simulink model "AEBTestBench"  (R2022b)
settings: Solver=ode45  StartTime=0.0  StopTime=inf  FixedStep=0.05  RelTol=1e-3
PostLoadFcn:
  | helperSLAEBSetup()
model workspace (MAT data in the model file):
  scenario : drivingScenario (value not decoded)
values from neighbouring files (symbols this model uses):
  actorsProfiles = rmfield(actorsProfiles,'MeshFaces')    [helperSLAEBSetup.m]
  egoActorID = egoVehicle.ActorID    [helperSLAEBSetup.m]
  egoRefPath = helperEgoRefPathCreator(scenario, egoActorID)    [helperSLAEBSetup.m]
  Ts = 0.05    [helperSLAEBSetup.m]
  v_set = norm(egoVehicle.Velocity)    [helperSLAEBSetup.m]
undefined symbols (not defined in the file or in its folder): cameraParams, driving, matlabshared, radarParams
libraries: drivingscenarioandsensors x3, simulink x2
CloseFcn:
  | helperSLAEBCleanup
settings Model: SILPILSystemUnderTest=refmodels  SnapshotInterval=5  PacingRate=0.220000  Creator=The MathWorks, Inc.  LastModifiedBy=yunuo
settings SolverCC: AlgebraicLoopSolver=TrustRegion  MinimalZcImpactIntegration=on  MaxZcPerStep=1
settings DataIOCC: SaveTime=off  ReturnWorkspaceOutputs=off
settings OptimizationCC: DefaultParameterBehavior=Inlined  InlineInvariantSignals=on  PassReuseOutputArgsAs=Individual arguments  ZeroExternalMemoryAtStartup=off  OptimizeBlockOrder=speed  EfficientTunableParamExpr=on
settings DebuggingCC: ParameterTunabilityLossMsg=error  UnconnectedInputMsg=warning  UnconnectedOutputMsg=warning  UnconnectedLineMsg=warning  PregeneratedLibrarySubsystemCodeDiagnostic=none  SFMachineParentedDataDiag=warning  ArithmeticOperatorsInVariantConditions=warning
settings HardwareCC: ProdLongLongMode=on
settings ModelReferenceCC: EnableRefExpFcnMdlSchedulingChecks=on  ModelReferenceNumInstancesAllowed=Single  PropagateVarSize=Only when enabling
settings SFSimCC: SimUseLocalCustomCode=off  CustomCodeUndefinedFunction=UseInterfaceOnly
settings RTWCC: Description=Embedded Coder  SystemTargetFile=ert.tlc  TemplateMakefile=ert_default_tmf  GenerateReport=on  RTWUseLocalCustomCode=off  BuildConfiguration=Faster Runs  IncludeHyperlinkInReport=on  LaunchReport=on  GenerateTraceInfo=on  GenerateTraceReport=on  GenerateTraceReportSl=on  GenerateTraceReportSf=on  GenerateTraceReportEml=on  GenerateCodeMetricsReport=on  DLArmComputeVersion=19.05
settings CodeAppCC: ForceParamTrailComments=on  IgnoreCustomStorageClasses=off  OperatorAnnotations=on  SimulinkDataObjDesc=on  SFDataObjDesc=on  CustomSymbolStrFcn=$N$M$F  InsertBlockDesc=on
settings ERTTargetCC: TargetLangStandard=C99 (ISO)  GenerateSampleERTMain=on  CombineSignalStateStructs=on  SuppressErrorStatus=on  InlinedParameterPlacement=NonHierarchical  RootIOFormat=Structure reference  RTWCAPISignals=on  ERTCustomFileTemplate=example_file_process.tlc

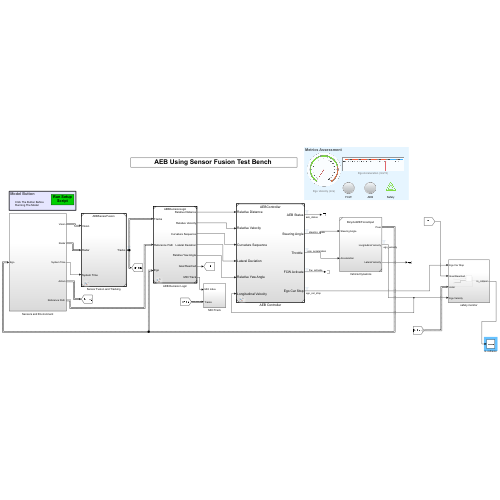
[thumbnail: Simulink's stored preview of the top-level diagram]
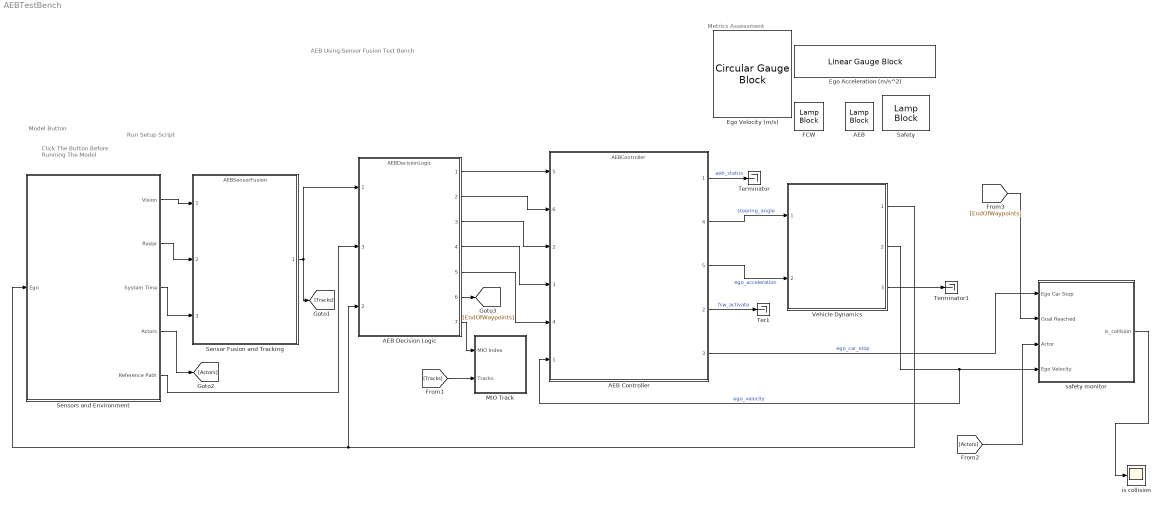
== system AEBTestBench ==
  note: Click The Button Before Running The Model
  note: Model Button
  note: AEB Using Sensor Fusion Test Bench
  note: Run Setup Script
  note: Metrics Assessment
  AEB : LampBlock  LabelPosition=Hide
  AEB Controller : ModelReference  ModelNameDialog=AEBController.slx  SimulationMode=Normal  CodeInterface=Top model  ModelReferenceVersion=5.0
      settings: PortSchema="{\"entries\":[{\"content\":{\"sides\":[{\"content\":{\"connectorIds\":[\"In5\",\"In6\",\"In2\",\"In3\",\"In4\",\"In1\"]},\"type\":\"ConnectorPlacement.EquallySpacedRectSide\",\"uuid\":\"48eb62e1-c687-4ccc-af1d-5db323c86b02\"},{\"content\":{\"connectorIds\":[\"Out1\",\"Out4\",\"Out5\",\"Out2\",\"Out3\"],\"side\":\"RIGHT\"},\"type\":\"ConnectorPlacement.EquallySpacedRectSide\",\"uuid\":\"cf0b79c1-cc3c-4144-ab0a-ade48c99ebae\"},{\"content\":{\"connectorIds\":[],\"side\":\"TOP\"},\"type\":\"ConnectorPlacement.EquallySpacedRectSide\",\"uuid\":\"b5029296-17a7-4a3b-9030-50c7482e3f67\"}]},\"type\":\"ConnectorPlacement.EquallySpacedConnector\",\"uuid\":\"17fe6146-247b-40c2-bc98-b1cbe9fc8f16\"}],\"packageUris\":[\"http://schema.mathworks.com/mf0/Connector/R2020b\"],\"version\":\"1.0\"}"
  AEB Decision Logic : ModelReference  ModelNameDialog=AEBDecisionLogic.slx  SimulationMode=Normal  CodeInterface=Top model  ModelReferenceVersion=5.1
      settings: PortSchema="{\"entries\":[{\"content\":{\"sides\":[{\"content\":{\"connectorIds\":[\"In1\",\"In3\",\"In2\"]},\"type\":\"ConnectorPlacement.EquallySpacedRectSide\",\"uuid\":\"e56e8f8b-a309-4236-958d-7c071b30483d\"},{\"content\":{\"connectorIds\":[\"Out1\",\"Out2\",\"Out3\",\"Out4\",\"Out5\",\"Out6\",\"Out7\"],\"side\":\"RIGHT\"},\"type\":\"ConnectorPlacement.EquallySpacedRectSide\",\"uuid\":\"786f45c2-22a8-47c8-9611-adc89b05d8ab\"},{\"content\":{\"connectorIds\":[],\"side\":\"TOP\"},\"type\":\"ConnectorPlacement.EquallySpacedRectSide\",\"uuid\":\"5bf649b4-ba14-4001-82ca-fb4560d0e6eb\"}]},\"type\":\"ConnectorPlacement.EquallySpacedConnector\",\"uuid\":\"abe3d890-2016-4578-afe8-a79cce07cd81\"}],\"packageUris\":[\"http://schema.mathworks.com/mf0/Connector/R2020b\"],\"version\":\"1.0\"}"
  Ego Acceleration (m/s^2) : LinearGaugeBlock  LabelPosition=Hide  ScaleMin=-9.8  ScaleMax=3  TickInterval=1
  Ego Velocity (m/s) : CircularGaugeBlock  LabelPosition=Hide  ScaleMax=20
  FCW : LampBlock  LabelPosition=Hide
  MIO Track : Subsystem
  Safety : LampBlock  LabelPosition=Hide  Icon=Hazards
  Sensor Fusion and Tracking : ModelReference  ModelNameDialog=AEBSensorFusion.slx  SimulationMode=Normal  CodeInterface=Top model  ModelReferenceVersion=5.2
  Sensors and Environment : Subsystem
  Ter1 : Terminator
  Terminator : Terminator
  Terminator1 : Terminator
  Vehicle Dynamics : Subsystem  ReferencedSubsystem=BicycleWithForceInput
  is collision : Scope
  safety monitor : Subsystem
  wires:
  AEB Controller/1 -> Terminator/1  "aeb_status"
  AEB Controller/2 -> Ter1/1  "fcw_activate"
  Vehicle Dynamics/1 -> Sensors and Environment/1(Ego), AEB Decision Logic/2
  Sensors and Environment/2(Radar) -> Sensor Fusion and Tracking/2
  Sensor Fusion and Tracking/1 -> AEB Decision Logic/1, [Tracks]
  Sensors and Environment/3(System Time) -> Sensor Fusion and Tracking/3
  Sensors and Environment/1(Vision) -> Sensor Fusion and Tracking/1
  AEB Decision Logic/5 -> AEB Controller/4
  AEB Decision Logic/4 -> AEB Controller/3
  AEB Decision Logic/3 -> AEB Controller/2
  AEB Decision Logic/1 -> AEB Controller/5
  AEB Decision Logic/2 -> AEB Controller/6
  AEB Decision Logic/6 -> [EndOfWaypoints]
  Sensors and Environment/4(Actors) -> [Actors]
  [Tracks] -> MIO Track/2(Tracks)
  AEB Decision Logic/7 -> MIO Track/1(MIO Index)
  Vehicle Dynamics/3 -> Terminator1/1
  AEB Controller/5 -> Vehicle Dynamics/2  "ego_acceleration"
  AEB Controller/4 -> Vehicle Dynamics/1  "steering_angle"
  Sensors and Environment/5("Reference Path ") -> AEB Decision Logic/3
  [Actors] -> safety monitor/3(Actor)
  [EndOfWaypoints] -> safety monitor/2(Goal Reached)
  AEB Controller/3 -> safety monitor/1(Ego Car Stop)  "ego_car_stop"
  Vehicle Dynamics/2 -> AEB Controller/1, safety monitor/4(Ego Velocity)  "ego_velocity"
  safety monitor/1(is_collision) -> is collision/1

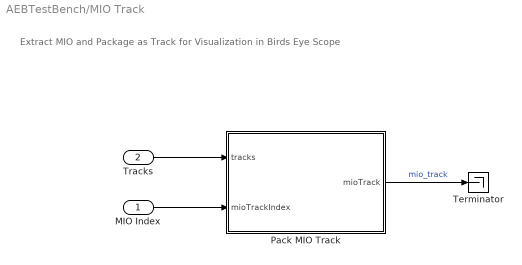
== system AEBTestBench/MIO Track ==
  note: Extract MIO and Package as Track for Visualization in Birds Eye Scope
  MIO Index : Inport
  Tracks : Inport  Port=2
  Pack MIO Track : MATLAB Function  TreatAsAtomicUnit=on
  Terminator : Terminator
  wires:
  Pack MIO Track/1(mioTrack) -> Terminator/1  "mio_track"
  Tracks/1 -> Pack MIO Track/1(tracks)
  MIO Index/1 -> Pack MIO Track/2(mioTrackIndex)

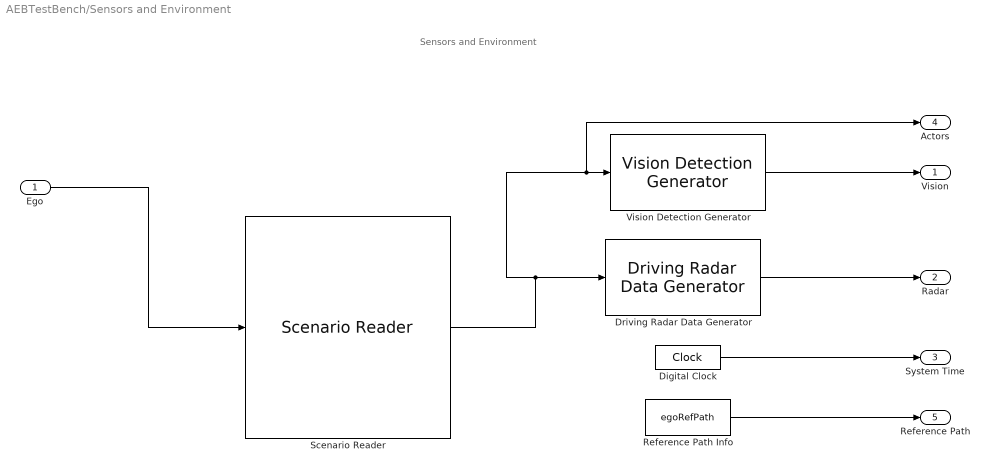
== system AEBTestBench/Sensors and Environment ==
  note: Sensors and Environment
  Ego : Inport
  Digital Clock : DigitalClock  SampleTime=Ts
  Driving Radar Data Generator : drivingscenarioandsensors/Driving Radar Data Generator  SensorIndex=2  UpdateRate=1/Ts  MountingLocation=[ 3.7, 0, 0.2 ]  MountingAngles=[0 0 0]  HasElevation=off  HasRangeRate=on  HasNoise=on  HasFalseAlarms=on  HasOcclusion=on  MaxNumReportsSource=Property  MaxNumReports=50  TargetReportFormat=Clustered detections  DetectionCoordinates=Body  TrackCoordinates=Body  BusNameSource=Property  BusName=BusRadar  AzimuthResolution=radarParams.azRes  ElevationResolution=5  RangeResolution=radarParams.rangeRes  RangeRateResolution=radarParams.rangeRateRes  AzimuthBiasFraction=0.1  ElevationBiasFraction=0.1  RangeBiasFraction=0.05  RangeRateBiasFraction=0.05  FieldOfView=[ radarParams.azFov, 5 ]  RangeLimits=[ 0, radarParams.radarRange ]  RangeRateLimits=[ -100, 100 ]  DetectionProbability=0.9  FalseAlarmRate=1e-06  ReferenceRange=100  ReferenceRCS=0  CenterFrequency=77e9  FilterInitializationFcn=initcvekf  ConfirmationThreshold=[2 3]  DeletionThreshold=[5 5]  InitialSeedSource=Repeatable  InitialSeed=0  UsedSeed=matlabshared.tracking.internal.SimulinkUtilities.seedManager(gcb)  ProfilesSource=From Scenario Reader block  ProfilesParameters=driving.internal.ActorProfilesRadarParameters  ProfilesExpression=struct('ClassID',0,'Length',4.7,'Width',1.8,'Height',1.4,'OriginOffset',[-1.35 0 0],'RCSPattern',[10 10;10 10],'RCSAzimuthAngles',[-180 180],'RCSElevationAngles',[-90 90])
  Reference Path Info : Constant  Value=egoRefPath  OutDataTypeStr=Bus: BusEgoRefPath  SampleTime=Ts
  Scenario Reader : drivingscenarioandsensors/Scenario Reader  ScenarioSource=From workspace  ScenarioFileName=AEB_CCRs_100overlap.mat  ScenarioVariableName=scenario  OutputCoordinateSystem=Vehicle coordinates  EgoVehicleSource=Input port  EgoVehicleActorID=egoActorID  OrientVehiclesOnRoad=on  OutputEgoVehiclePose=off  OutputEgoVehicleState=off  SampleTime=Ts  LaneBoundaryOutput=None  LaneBoundaryDistance=0:0.5:9.5  LaneBoundaryLocation=Center of lane markings  BusNameSource=Auto  BusName=BusActors  BusNumActorsSource=Scenario  BusNumActors=100  BusName2Source=Auto  BusName2=BusLaneBoundaries  BusNumLaneBoundariesSource=Scenario  BusNumLaneBoundaries=10  BusName3Source=Auto  BusName3=BusEgoActor  BusName4Source=Auto  BusName4=BusEgoState  ShowCoordinateLabels=on  SimulateUsing=Interpreted execution
  Vision Detection Generator : drivingscenarioandsensors/Vision Detection Generator  SensorIndex=1  DetectorOutput=Objects only  UpdateInterval=Ts  LaneUpdateInterval=Ts  SensorLocation=[ 2.1, 0 ]  Height=1.1  Yaw=0  Pitch=cameraParams.pitchAngle  Roll=0  BusNameSource=Property  BusName=BusVision  BusName2Source=Auto  BusName2=BusLaneDetections  MaxNumDetectionsSource=Property  MaxNumDetections=20  MaxNumLanesSource=Property  MaxNumLanes=30  DetectionCoordinates=Ego Cartesian  SimulateUsing=Interpreted execution  MaxRange=cameraParams.cameraRange  BoundingBoxAccuracy=5  ProcessNoiseIntensity=5  MaxSpeed=50  MaxAllowedOcclusion=0.5  MinObjectImageSize=[ 15, 15 ]  DetectionProbability=0.9  FalsePositivesPerImage=0.1  MinLaneImageSize=[ 20, 5 ]  LaneBoundaryAccuracy=3  HasNoise=on  InitialSeedSource=Repeatable  InitialSeed=0  UsedSeed=driving.internal.SimulinkUtilities.seedManager(gcb)  ActorProfilesSource=From Scenario Reader block  ActorProfilesParameters=driving.internal.ActorProfilesParameters  ActorProfilesExpression=struct( 'ClassID', 0, 'Length', 4.7, 'Width', 1.8, 'Height', 1.4, 'OriginOffset', [ -1.35, 0, 0 ] )  Intrinsics=driving.internal.cameraIntrinsics('FocalLength',cameraParams.focalLength,'PrincipalPoint',cameraParams.principalPoint,'ImageSize',cameraParams.imageSize)
  Vision : Outport  VectorParamsAs1DForOutWhenUnconnected=off
  Radar : Outport  Port=2  OutDataTypeStr=Bus: BusRadar  VectorParamsAs1DForOutWhenUnconnected=off
  System Time : Outport  Port=3  VectorParamsAs1DForOutWhenUnconnected=off
  Actors : Outport  Port=4
  "Reference Path " : Outport  Port=5
  wires:
  Vision Detection Generator/1 -> Vision/1
  Ego/1 -> Scenario Reader/1
  Digital Clock/1 -> System Time/1
  Driving Radar Data Generator/1 -> Radar/1
  Scenario Reader/1 -> Actors/1, Vision Detection Generator/1, Driving Radar Data Generator/1
  Reference Path Info/1 -> "Reference Path "/1

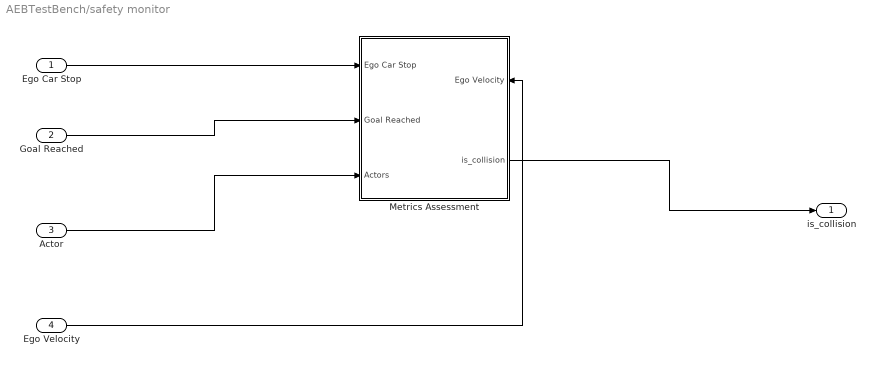
== system AEBTestBench/safety monitor ==
  Ego Car Stop : Inport
  Goal Reached : Inport  Port=2
  Actor : Inport  Port=3
  Ego Velocity : Inport  Port=4
  Metrics Assessment : Subsystem
      settings: PortSchema="{\"entries\":[{\"content\":{\"sides\":[{\"content\":{\"connectorIds\":[\"In1\",\"In2\",\"In3\"]},\"type\":\"ConnectorPlacement.EquallySpacedRectSide\",\"uuid\":\"d600d027-9714-4589-bd74-ff85c373770c\"},{\"content\":{\"connectorIds\":[\"In4\",\"Out1\"],\"side\":\"RIGHT\"},\"type\":\"ConnectorPlacement.EquallySpacedRectSide\",\"uuid\":\"c68a0d3a-3a81-49cd-ba70-f2de3f1a882f\"},{\"content\":{\"connectorIds\":[],\"side\":\"TOP\"},\"type\":\"ConnectorPlacement.EquallySpacedRectSide\",\"uuid\":\"d9b15fac-7ed3-4474-96f3-d7b693286234\"},{\"content\":{\"connectorIds\":[],\"side\":\"BOTTOM\"},\"type\":\"ConnectorPlacement.EquallySpacedRectSide\",\"uuid\":\"00c5a332-b546-4dc5-aa31-259f1868ab67\"}]},\"type\":\"ConnectorPlacement.EquallySpacedConnector\",\"uuid\":\"e6d068d7-d2df-4de9-99aa-2a189a2c2730\"}],\"packageUris\":[\"http://schema.mathworks.com/mf0/Connector/R2020b\"],\"version\":\"1.0\"}"
  is_collision : Outport
  wires:
  Ego Car Stop/1 -> Metrics Assessment/1(Ego Car Stop)
  Goal Reached/1 -> Metrics Assessment/2(Goal Reached)
  Actor/1 -> Metrics Assessment/3(Actors)
  Ego Velocity/1 -> Metrics Assessment/4(Ego Velocity)
  Metrics Assessment/1(is_collision) -> is_collision/1

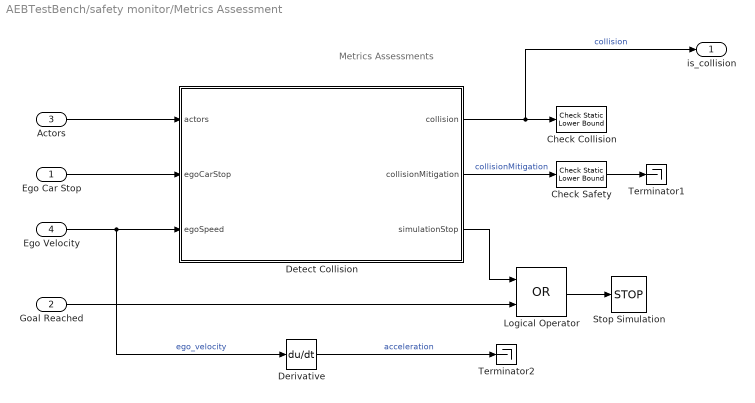
== system AEBTestBench/safety monitor/Metrics Assessment ==
  note: Metrics Assessments
  Ego Car Stop : Inport
  Goal Reached : Inport  Port=2
  Actors : Inport  Port=3
  Ego Velocity : Inport  Port=4
  Check Collision : simulink/Model Verification/Check Static  Lower Bound  Description=0 <= u  min=0  min_included=on  enabled=on  stopWhenAssertionFail=off  export=off  icon=graphic
  Check Safety : simulink/Model Verification/Check Static  Lower Bound  Description=safetyGoal <= u  min=safetyGoal  min_included=on  enabled=on  stopWhenAssertionFail=off  export=on  icon=graphic
  Derivative : Derivative
  Detect Collision : MATLAB Function  TreatAsAtomicUnit=on  mask(Detect Collision){vehicleProfiles=actorsProfiles, setSpeed=v_set, egoActorID=egoActorID}
      mask prompts: vehicleProfiles "Vehicle profiles"; setSpeed "Set Speed"; egoActorID "Ego Actor ID"
      mask help:
      | Detect collision between ego and target vehicles.
      | Vehicle profiles is expected to be the struture returned by the actorProfiles method of a drivingScenerio object.
      settings: AttributesFormatString=|
      | ------------------------------------------
      | vehicleProfiles = %<vehicleProfiles>
  Logical Operator : Logic  Operator=OR  AllPortsSameDT=off  OutDataTypeStr=boolean
  Stop Simulation : Stop
  Terminator1 : Terminator
  Terminator2 : Terminator
  is_collision : Outport
  wires:
  Ego Car Stop/1 -> Detect Collision/2(egoCarStop)
  Derivative/1 -> Terminator2/1  "acceleration"
  Ego Velocity/1 -> Derivative/1, Detect Collision/3(egoSpeed)  "ego_velocity"
  Actors/1 -> Detect Collision/1(actors)
  Detect Collision/1(collision) -> is_collision/1, Check Collision/1  "collision"
  Detect Collision/2(collisionMitigation) -> Check Safety/1  "collisionMitigation"
  Goal Reached/1 -> Logical Operator/2
  Logical Operator/1 -> Stop Simulation/1
  Detect Collision/3(simulationStop) -> Logical Operator/1
  Check Safety/1 -> Terminator1/1

== matlab function AEBTestBench/safety monitor/Metrics Assessment/Detect Collision ==
  data: actors input; collision output; vehicleProfiles parameter; egoCarStop input; collisionMitigation output; simulationStop output; setSpeed parameter; egoSpeed input double; egoActorID parameter
function [collision, collisionMitigation, simulationStop] = detectCollision(actors, vehicleProfiles, egoCarStop, setSpeed, egoSpeed, egoActorID)

% Associate on-path MATLAB function
coder.extrinsic('helperSLDetectVehicleCollision', 'warning');

% Assign default value to define output data type
collision = false;

% Call on-path MATLAB function
collision = helperSLDetectVehicleCollision(actors.Actors, vehicleProfiles, egoActorID = egoActorID);

if egoCarStop==true && collision==false
    collisionMitigation = 100.0; % Full collision avoidance = 100% collision migitation
elseif collision==true % collision detection
    collisionMitigation  = 100*(setSpeed-egoSpeed)/setSpeed; % calculate collision migitation
else
    collisionMitigation = 100.0; % neither collision nor ego car stop
end 

% if collision==true
%    error('Simulation stopped because of collision');
% end

if egoCarStop==true || collision==true
    simulationStop = true;
else
    simulationStop = false;
end

== matlab function AEBTestBench/MIO Track/Pack MIO Track ==
  data: tracks input; mioTrack output Bus: BusMultiObjectTracker1; mioTrackIndex input
function mioTrack = fcn(tracks, mioTrackIndex)
% Extract MIO track and package for visualization in Birds Eye Scope

mioTrack = tracks;

if mioTrackIndex > 0
    % First track represents MIO
    mioTrack.NumTracks = 1;
    mioTrack.Tracks(1) = tracks.Tracks(mioTrackIndex);
else
    % No valid MIO track
    mioTrack.NumTracks = 0;
end
